simulink library "VACLib"  (R2022b)
settings: Solver=VariableStepAuto  StartTime=0.0  StopTime=10.0  RelTol=1e-3
settings Model: Creator=KarlO  LastModifiedBy=JMESSING

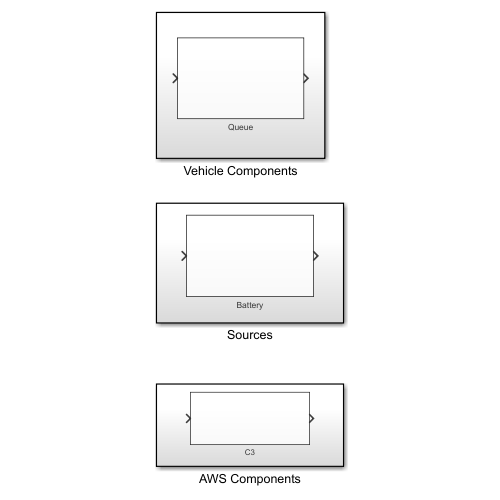
[thumbnail: Simulink's stored preview of the top-level diagram]
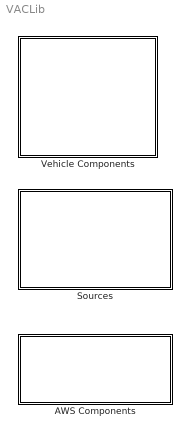
== system VACLib ==
  AWS Components : Subsystem
  Sources : Subsystem
  Vehicle Components : Subsystem

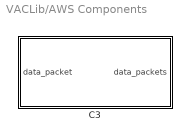
== system VACLib/AWS Components ==
  C3 : MATLAB Function  TreatAsAtomicUnit=on

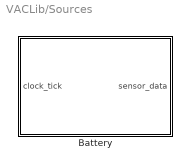
== system VACLib/Sources ==
  Battery : MATLAB Function  TreatAsAtomicUnit=on  mask{sensor_data_size=8}
      mask prompts: sensor_data_size "Sensor Data Size (kB)"

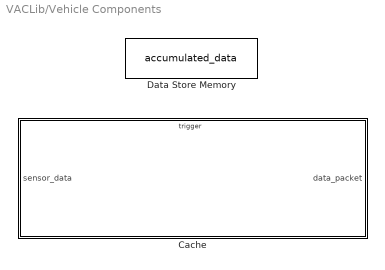
== system VACLib/Vehicle Components ==
  Cache : MATLAB Function  TreatAsAtomicUnit=on  mask{cache_size=0}
      mask prompts: cache_size "Cache Size"
  Data Store Memory : DataStoreMemory  DataStoreName=accumulated_data  WriteAfterWriteMsg=warning  ShowAdditionalParam=off

== matlab function VACLib/Vehicle Components/Cache ==
  data: sensor_data input double; data_packet output double; cache_size parameter; accumulated_data data_store_memory
  events: trigger input EITHER_EDGE_EVENT
function data_packet  = cache(sensor_data, cache_size)

global accumulated_data;
accumulated_data = accumulated_data + sensor_data;
if accumulated_data >= cache_size
    data_packet = accumulated_data;
    accumulated_data = 0;
else
    data_packet = 0;
end

== matlab function VACLib/AWS Components/C3 ==
  data: data_packet input; data_packets output; consistency parameter
function data_packets = C3(data_packet, consistency)
%Consistency should be 0, 1 or 2, and corresponds to different consistency
%types
tic;
global total_time;
switch consistency
    case 0
        data_packets = data_packet / 8 / 100;
        delay_time = 10;
        total_time = toc + delay_time;
    case 1
        data_packets =  data_packet / 8 / 50;
        delay_time = 5;
        total_time = toc + delay_time;
    case 2
        data_packets =  data_packet / 8 / 10;
        delay_time = 1;
        total_time = toc + delay_time;
    otherwise
        error('Invalid consistency type');
end
end

== matlab function VACLib/Sources/Battery ==
  data: clock_tick input; sensor_data output; sensor_data_size parameter
function sensor_data = battery(clock_tick, sensor_data_size)

sensor_data = clock_tick * sensor_data_size;
